simulink model "case4"  (R2024b)
settings: Solver=FixedStepAuto  StartTime=0  StopTime=1  FixedStep=1e-7  RelTol=1e-3
values from neighbouring files (symbols this model uses):
  SG_D_1_D = 0.01056    [IEEE9_case_parameters.m]    (also in case1_parameters.m; case2_parameters.m; case3_parameters.m; case4_parameters.m)
  SG_D_1_EnableSaturation = 0    [IEEE9_case_parameters.m]    (also in case1_parameters.m; case2_parameters.m; case3_parameters.m; case4_parameters.m)
  SG_D_1_f0 = 60    [IEEE9_case_parameters.m]    (also in case1_parameters.m; case2_parameters.m; case3_parameters.m; case4_parameters.m)
  SG_D_1_H = 7.5    [IEEE9_case_parameters.m]    (also in case1_parameters.m; case2_parameters.m; case3_parameters.m; case4_parameters.m)
  SG_D_1_K_A = 20    [IEEE9_case_parameters.m]    (also in case1_parameters.m; case2_parameters.m; case3_parameters.m; case4_parameters.m)
  SG_D_1_K_E = 1.000000e+1    (= 10)    [IEEE9_case_parameters.m]    (also in case1_parameters.m; case2_parameters.m; case3_parameters.m; case4_parameters.m)
  SG_D_1_K_F = 2.363    [IEEE9_case_parameters.m]    (also in case1_parameters.m; case2_parameters.m; case3_parameters.m; case4_parameters.m)
  SG_D_1_K_s = 0.5    [IEEE9_case_parameters.m]    (also in case1_parameters.m = 5; case2_parameters.m = 5; case3_parameters.m = 5; case4_parameters.m = 5)
  SG_D_1_R_a = 0.001088    [IEEE9_case_parameters.m]    (also in case1_parameters.m; case2_parameters.m; case3_parameters.m; case4_parameters.m)
  SG_D_1_S_A = 1    [IEEE9_case_parameters.m]    (also in case1_parameters.m; case2_parameters.m; case3_parameters.m; case4_parameters.m)
  SG_D_1_S_B = 0.103    [IEEE9_case_parameters.m]    (also in case1_parameters.m; case2_parameters.m; case3_parameters.m; case4_parameters.m)
  SG_D_1_S_N = 10.659857    [IEEE9_case_parameters.m]    (also in case1_parameters.m; case2_parameters.m; case3_parameters.m; case4_parameters.m)
  SG_D_1_SpeedPara = 200    [IEEE9_case_parameters.m]    (also in case1_parameters.m; case2_parameters.m; case3_parameters.m; case4_parameters.m)
  SG_D_1_T_0 = 0.720173    [IEEE9_case_parameters.m]    (also in case1_parameters.m = 0.755522; case2_parameters.m = 0.808931; case3_parameters.m = 0.869402; case4_parameters.m = 0.729316)
  SG_D_1_T_1 = 0.3    [IEEE9_case_parameters.m]    (also in case1_parameters.m; case2_parameters.m; case3_parameters.m; case4_parameters.m)
  SG_D_1_T_2 = 0.05    [IEEE9_case_parameters.m]    (also in case1_parameters.m; case2_parameters.m; case3_parameters.m; case4_parameters.m)
  SG_D_1_T_3 = 0.02    [IEEE9_case_parameters.m]    (also in case1_parameters.m; case2_parameters.m; case3_parameters.m; case4_parameters.m)
  SG_D_1_T_4 = 0.005    [IEEE9_case_parameters.m]    (also in case1_parameters.m; case2_parameters.m; case3_parameters.m; case4_parameters.m)
  SG_D_1_T_A = 0.02    [IEEE9_case_parameters.m]    (also in case1_parameters.m; case2_parameters.m; case3_parameters.m; case4_parameters.m)
  SG_D_1_T_dd = 8.000000e+0    (= 8)    [IEEE9_case_parameters.m]    (also in case1_parameters.m; case2_parameters.m; case3_parameters.m; case4_parameters.m)
  SG_D_1_T_ddd = 0.04    [IEEE9_case_parameters.m]    (also in case1_parameters.m; case2_parameters.m; case3_parameters.m; case4_parameters.m)
  SG_D_1_T_E = 0.314    [IEEE9_case_parameters.m]    (also in case1_parameters.m; case2_parameters.m; case3_parameters.m; case4_parameters.m)
  SG_D_1_T_F = 0.35    [IEEE9_case_parameters.m]    (also in case1_parameters.m; case2_parameters.m; case3_parameters.m; case4_parameters.m)
  SG_D_1_T_qd = 0.8    [IEEE9_case_parameters.m]    (also in case1_parameters.m; case2_parameters.m; case3_parameters.m; case4_parameters.m)
  SG_D_1_T_qdd = 0.02    [IEEE9_case_parameters.m]    (also in case1_parameters.m; case2_parameters.m; case3_parameters.m; case4_parameters.m)
  SG_D_1_T_speed = 0.1    [IEEE9_case_parameters.m]    (also in case1_parameters.m = 200; case2_parameters.m = 200; case3_parameters.m = 200; case4_parameters.m = 200)
  SG_D_1_T_w = 0.5    [IEEE9_case_parameters.m]    (also in case1_parameters.m; case2_parameters.m; case3_parameters.m; case4_parameters.m)
  SG_D_1_V_ref = 1.990276    [IEEE9_case_parameters.m]    (also in case1_parameters.m = 2.042296; case2_parameters.m = 2.051388; case3_parameters.m = 2.089584; case4_parameters.m = 2.01845)
  SG_D_1_w_ref = 376.991118    [IEEE9_case_parameters.m]    (also in case1_parameters.m; case2_parameters.m; case3_parameters.m; case4_parameters.m)
  SG_D_1_wb = 6.000000e+1    (= 60)    [IEEE9_case_parameters.m]    (also in case1_parameters.m; case2_parameters.m; case3_parameters.m; case4_parameters.m)
  SG_D_1_x_d = 1.9    [IEEE9_case_parameters.m]    (also in case1_parameters.m; case2_parameters.m; case3_parameters.m; case4_parameters.m)
  SG_D_1_x_dd = 0.302    [IEEE9_case_parameters.m]    (also in case1_parameters.m; case2_parameters.m; case3_parameters.m; case4_parameters.m)
  SG_D_1_x_ddd = 0.204    [IEEE9_case_parameters.m]    (also in case1_parameters.m; case2_parameters.m; case3_parameters.m; case4_parameters.m)
  SG_D_1_x_l = 0.05    [IEEE9_case_parameters.m]    (also in case1_parameters.m; case2_parameters.m; case3_parameters.m; case4_parameters.m)
  SG_D_1_x_q = 1.3    [IEEE9_case_parameters.m]    (also in case1_parameters.m; case2_parameters.m; case3_parameters.m; case4_parameters.m)
  SG_D_1_x_qd = 0.5    [IEEE9_case_parameters.m]    (also in case1_parameters.m; case2_parameters.m; case3_parameters.m; case4_parameters.m)
  SG_D_1_x_qdd = 0.3    [IEEE9_case_parameters.m]    (also in case1_parameters.m; case2_parameters.m; case3_parameters.m; case4_parameters.m)
  SG_D_2_D = 0.02    [IEEE9_case_parameters.m]    (also in case1_parameters.m; case2_parameters.m; case3_parameters.m; case4_parameters.m)
  SG_D_2_EnableSaturation = 0    [IEEE9_case_parameters.m]    (also in case1_parameters.m; case2_parameters.m; case3_parameters.m; case4_parameters.m)
  SG_D_2_f0 = 60    [IEEE9_case_parameters.m]    (also in case1_parameters.m; case2_parameters.m; case3_parameters.m; case4_parameters.m)
  SG_D_2_H = 8.000000e+0    (= 8)    [IEEE9_case_parameters.m]    (also in case1_parameters.m; case2_parameters.m; case3_parameters.m; case4_parameters.m)
  SG_D_2_K_A = 20    [IEEE9_case_parameters.m]    (also in case1_parameters.m; case2_parameters.m; case3_parameters.m; case4_parameters.m)
  SG_D_2_K_E = 1.000000e+1    (= 10)    [IEEE9_case_parameters.m]    (also in case1_parameters.m; case2_parameters.m; case3_parameters.m; case4_parameters.m)
  SG_D_2_K_F = 2.363    [IEEE9_case_parameters.m]    (also in case1_parameters.m; case2_parameters.m; case3_parameters.m; case4_parameters.m)
  SG_D_2_K_s = 0.5    [IEEE9_case_parameters.m]    (also in case1_parameters.m = 4; case2_parameters.m = 4; case3_parameters.m = 4; case4_parameters.m = 4)
  SG_D_2_R_a = 0.001088    [IEEE9_case_parameters.m]    (also in case1_parameters.m; case2_parameters.m; case3_parameters.m; case4_parameters.m)
  SG_D_2_S_A = 1    [IEEE9_case_parameters.m]    (also in case1_parameters.m; case2_parameters.m; case3_parameters.m; case4_parameters.m)
  SG_D_2_S_B = 0.103    [IEEE9_case_parameters.m]    (also in case1_parameters.m; case2_parameters.m; case3_parameters.m; case4_parameters.m)
  SG_D_2_S_N = 10.659857    [IEEE9_case_parameters.m]    (also in case1_parameters.m; case2_parameters.m; case3_parameters.m; case4_parameters.m)
  SG_D_2_SpeedPara = 200    [IEEE9_case_parameters.m]    (also in case1_parameters.m; case2_parameters.m; case3_parameters.m; case4_parameters.m)
  SG_D_2_T_0 = 1.632913    [IEEE9_case_parameters.m]    (also in case1_parameters.m = 1.632925; case2_parameters.m = 1.632915; case3_parameters.m = 1.632914; case4_parameters.m = 1.632927)
  SG_D_2_T_1 = 0.2    [IEEE9_case_parameters.m]    (also in case1_parameters.m; case2_parameters.m; case3_parameters.m; case4_parameters.m)
  SG_D_2_T_2 = 0.05    [IEEE9_case_parameters.m]    (also in case1_parameters.m; case2_parameters.m; case3_parameters.m; case4_parameters.m)
  SG_D_2_T_3 = 0.02    [IEEE9_case_parameters.m]    (also in case1_parameters.m; case2_parameters.m; case3_parameters.m; case4_parameters.m)
  SG_D_2_T_4 = 0.005    [IEEE9_case_parameters.m]    (also in case1_parameters.m; case2_parameters.m; case3_parameters.m; case4_parameters.m)
  SG_D_2_T_A = 0.02    [IEEE9_case_parameters.m]    (also in case1_parameters.m; case2_parameters.m; case3_parameters.m; case4_parameters.m)
  SG_D_2_T_dd = 7.9    [IEEE9_case_parameters.m]    (also in case1_parameters.m; case2_parameters.m; case3_parameters.m; case4_parameters.m)
  SG_D_2_T_ddd = 0.04    [IEEE9_case_parameters.m]    (also in case1_parameters.m; case2_parameters.m; case3_parameters.m; case4_parameters.m)
  SG_D_2_T_E = 0.314    [IEEE9_case_parameters.m]    (also in case1_parameters.m; case2_parameters.m; case3_parameters.m; case4_parameters.m)
  SG_D_2_T_F = 0.35    [IEEE9_case_parameters.m]    (also in case1_parameters.m; case2_parameters.m; case3_parameters.m; case4_parameters.m)
  SG_D_2_T_qd = 0.8    [IEEE9_case_parameters.m]    (also in case1_parameters.m; case2_parameters.m; case3_parameters.m; case4_parameters.m)
  SG_D_2_T_qdd = 0.015    [IEEE9_case_parameters.m]    (also in case1_parameters.m; case2_parameters.m; case3_parameters.m; case4_parameters.m)
  SG_D_2_T_speed = 0.1    [IEEE9_case_parameters.m]    (also in case1_parameters.m = 150; case2_parameters.m = 150; case3_parameters.m = 150; case4_parameters.m = 150)
  SG_D_2_T_w = 0.35    [IEEE9_case_parameters.m]    (also in case1_parameters.m; case2_parameters.m; case3_parameters.m; case4_parameters.m)
  SG_D_2_V_ref = 2.58547    [IEEE9_case_parameters.m]    (also in case1_parameters.m = 2.597896; case2_parameters.m = 2.587136; case3_parameters.m = 2.586042; case4_parameters.m = 2.599679)
  SG_D_2_w_ref = 376.991118    [IEEE9_case_parameters.m]    (also in case1_parameters.m; case2_parameters.m; case3_parameters.m; case4_parameters.m)
  SG_D_2_wb = 6.000000e+1    (= 60)    [IEEE9_case_parameters.m]    (also in case1_parameters.m; case2_parameters.m; case3_parameters.m; case4_parameters.m)
  SG_D_2_x_d = 1.8    [IEEE9_case_parameters.m]    (also in case1_parameters.m; case2_parameters.m; case3_parameters.m; case4_parameters.m)
  SG_D_2_x_dd = 0.302    [IEEE9_case_parameters.m]    (also in case1_parameters.m; case2_parameters.m; case3_parameters.m; case4_parameters.m)
  SG_D_2_x_ddd = 0.204    [IEEE9_case_parameters.m]    (also in case1_parameters.m; case2_parameters.m; case3_parameters.m; case4_parameters.m)
  SG_D_2_x_l = 0.05    [IEEE9_case_parameters.m]    (also in case1_parameters.m; case2_parameters.m; case3_parameters.m; case4_parameters.m)
  SG_D_2_x_q = 1.25    [IEEE9_case_parameters.m]    (also in case1_parameters.m; case2_parameters.m; case3_parameters.m; case4_parameters.m)
  SG_D_2_x_qd = 0.5    [IEEE9_case_parameters.m]    (also in case1_parameters.m; case2_parameters.m; case3_parameters.m; case4_parameters.m)
  SG_D_2_x_qdd = 0.3    [IEEE9_case_parameters.m]    (also in case1_parameters.m; case2_parameters.m; case3_parameters.m; case4_parameters.m)
  SG_D_3_D = 0.02    [IEEE9_case_parameters.m]    (also in case1_parameters.m; case2_parameters.m; case3_parameters.m; case4_parameters.m)
  SG_D_3_EnableSaturation = 0    [IEEE9_case_parameters.m]    (also in case1_parameters.m; case2_parameters.m; case3_parameters.m; case4_parameters.m)
  SG_D_3_f0 = 60    [IEEE9_case_parameters.m]    (also in case1_parameters.m; case2_parameters.m; case3_parameters.m; case4_parameters.m)
  SG_D_3_H = 7.7    [IEEE9_case_parameters.m]    (also in case1_parameters.m; case2_parameters.m; case3_parameters.m; case4_parameters.m)
  SG_D_3_K_A = 20    [IEEE9_case_parameters.m]    (also in case1_parameters.m; case2_parameters.m; case3_parameters.m; case4_parameters.m)
  SG_D_3_K_E = 1.000000e+1    (= 10)    [IEEE9_case_parameters.m]    (also in case1_parameters.m; case2_parameters.m; case3_parameters.m; case4_parameters.m)
  SG_D_3_K_F = 2.363    [IEEE9_case_parameters.m]    (also in case1_parameters.m; case2_parameters.m; case3_parameters.m; case4_parameters.m)
  SG_D_3_K_s = 0.2    [IEEE9_case_parameters.m]    (also in case1_parameters.m = 2; case2_parameters.m = 2; case3_parameters.m = 2; case4_parameters.m = 2)
  SG_D_3_R_a = 0.001088    [IEEE9_case_parameters.m]    (also in case1_parameters.m; case2_parameters.m; case3_parameters.m; case4_parameters.m)
  SG_D_3_S_A = 1    [IEEE9_case_parameters.m]    (also in case1_parameters.m; case2_parameters.m; case3_parameters.m; case4_parameters.m)
  SG_D_3_S_B = 0.103    [IEEE9_case_parameters.m]    (also in case1_parameters.m; case2_parameters.m; case3_parameters.m; case4_parameters.m)
  SG_D_3_S_N = 10.659857    [IEEE9_case_parameters.m]    (also in case1_parameters.m; case2_parameters.m; case3_parameters.m; case4_parameters.m)
  SG_D_3_SpeedPara = 200    [IEEE9_case_parameters.m]    (also in case1_parameters.m; case2_parameters.m; case3_parameters.m; case4_parameters.m)
  SG_D_3_T_0 = 0.850788    [IEEE9_case_parameters.m]    (also in case1_parameters.m = 0.850786; case2_parameters.m = 0.850787; case3_parameters.m; case4_parameters.m = 0.850786)
  SG_D_3_T_1 = 0.2    [IEEE9_case_parameters.m]    (also in case1_parameters.m; case2_parameters.m; case3_parameters.m; case4_parameters.m)
  SG_D_3_T_2 = 0.05    [IEEE9_case_parameters.m]    (also in case1_parameters.m; case2_parameters.m; case3_parameters.m; case4_parameters.m)
  SG_D_3_T_3 = 0.02    [IEEE9_case_parameters.m]    (also in case1_parameters.m; case2_parameters.m; case3_parameters.m; case4_parameters.m)
  SG_D_3_T_4 = 0.005    [IEEE9_case_parameters.m]    (also in case1_parameters.m; case2_parameters.m; case3_parameters.m; case4_parameters.m)
  SG_D_3_T_A = 0.02    [IEEE9_case_parameters.m]    (also in case1_parameters.m; case2_parameters.m; case3_parameters.m; case4_parameters.m)
  SG_D_3_T_dd = 8.1    [IEEE9_case_parameters.m]    (also in case1_parameters.m; case2_parameters.m; case3_parameters.m; case4_parameters.m)
  SG_D_3_T_ddd = 0.04    [IEEE9_case_parameters.m]    (also in case1_parameters.m; case2_parameters.m; case3_parameters.m; case4_parameters.m)
  SG_D_3_T_E = 0.314    [IEEE9_case_parameters.m]    (also in case1_parameters.m; case2_parameters.m; case3_parameters.m; case4_parameters.m)
  SG_D_3_T_F = 0.35    [IEEE9_case_parameters.m]    (also in case1_parameters.m; case2_parameters.m; case3_parameters.m; case4_parameters.m)
  SG_D_3_T_qd = 0.8    [IEEE9_case_parameters.m]    (also in case1_parameters.m; case2_parameters.m; case3_parameters.m; case4_parameters.m)
  SG_D_3_T_qdd = 0.015    [IEEE9_case_parameters.m]    (also in case1_parameters.m; case2_parameters.m; case3_parameters.m; case4_parameters.m)
  SG_D_3_T_speed = 0.1    [IEEE9_case_parameters.m]    (also in case1_parameters.m = 180; case2_parameters.m = 180; case3_parameters.m = 180; case4_parameters.m = 180)
  SG_D_3_T_w = 0.4    [IEEE9_case_parameters.m]    (also in case1_parameters.m; case2_parameters.m; case3_parameters.m; case4_parameters.m)
  SG_D_3_V_ref = 1.892727    [IEEE9_case_parameters.m]    (also in case1_parameters.m = 1.906439; case2_parameters.m = 1.895535; case3_parameters.m = 1.892105; case4_parameters.m = 1.906598)
  SG_D_3_w_ref = 376.991118    [IEEE9_case_parameters.m]    (also in case1_parameters.m; case2_parameters.m; case3_parameters.m; case4_parameters.m)
  SG_D_3_wb = 6.000000e+1    (= 60)    [IEEE9_case_parameters.m]    (also in case1_parameters.m; case2_parameters.m; case3_parameters.m; case4_parameters.m)
  SG_D_3_x_d = 1.85    [IEEE9_case_parameters.m]    (also in case1_parameters.m; case2_parameters.m; case3_parameters.m; case4_parameters.m)
  SG_D_3_x_dd = 0.302    [IEEE9_case_parameters.m]    (also in case1_parameters.m; case2_parameters.m; case3_parameters.m; case4_parameters.m)
  SG_D_3_x_ddd = 0.204    [IEEE9_case_parameters.m]    (also in case1_parameters.m; case2_parameters.m; case3_parameters.m; case4_parameters.m)
  SG_D_3_x_l = 0.05    [IEEE9_case_parameters.m]    (also in case1_parameters.m; case2_parameters.m; case3_parameters.m; case4_parameters.m)
  SG_D_3_x_q = 1.2    [IEEE9_case_parameters.m]    (also in case1_parameters.m; case2_parameters.m; case3_parameters.m; case4_parameters.m)
  SG_D_3_x_qd = 0.5    [IEEE9_case_parameters.m]    (also in case1_parameters.m; case2_parameters.m; case3_parameters.m; case4_parameters.m)
  SG_D_3_x_qdd = 0.3    [IEEE9_case_parameters.m]    (also in case1_parameters.m; case2_parameters.m; case3_parameters.m; case4_parameters.m)
(part 1 of 12)
settings Model: Creator=Greg  LastModifiedBy=Greg

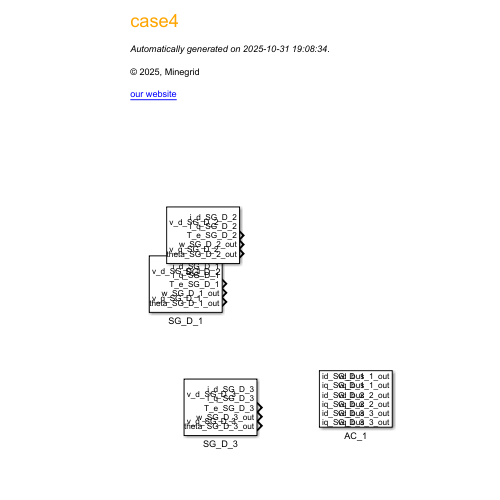
[thumbnail: Simulink's stored preview of the top-level diagram]
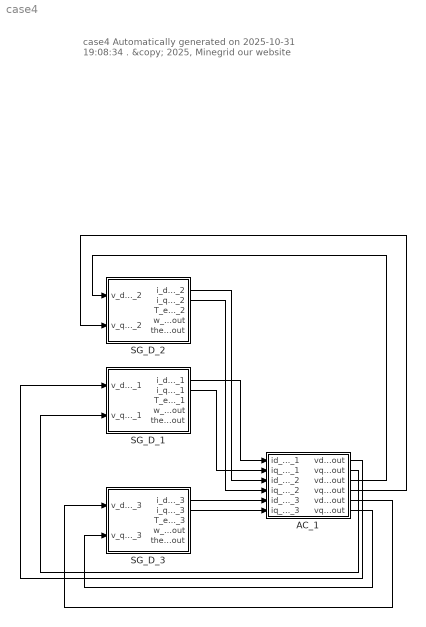
== system case4 ==
  note: case4
      | Automatically generated on 2025-10-31 19:08:34 .
      | &copy; 2025, Minegrid
      | our website
  AC_1 : Subsystem  mask(AC_1){}
      mask help: Parameters Interface of AC_1
  SG_D_1 : Subsystem  mask(SG_D_1){T_0=SG_D_1_T_0, w_ref=SG_D_1_w_ref, V_ref=SG_D_1_V_ref, x_d=SG_D_1_x_d, x_dd=SG_D_1_x_dd, x_ddd=SG_D_1_x_ddd, x_q=SG_D_1_x_q, x_qd=SG_D_1_x_qd, x_qdd=SG_D_1_x_qdd, x_l=SG_D_1_x_l, R_a=SG_D_1_R_a, T_dd=SG_D_1_T_dd, T_ddd=SG_D_1_T_ddd, T_qd=SG_D_1_T_qd, T_qdd=SG_D_1_T_qdd, H=SG_D_1_H, D=SG_D_1_D, SpeedPara=SG_D_1_SpeedPara, K_A=SG_D_1_K_A, EnableSaturation=SG_D_1_EnableSaturation, f0=SG_D_1_f0, T_speed=SG_D_1_T_speed, T_E=SG_D_1_T_E, T_A=SG_D_1_T_A, T_F=SG_D_1_T_F, K_E=SG_D_1_K_E, K_F=SG_D_1_K_F, K_s=SG_D_1_K_s, T_1=SG_D_1_T_1, T_2=SG_D_1_T_2, T_3=SG_D_1_T_3, T_4=SG_D_1_T_4, T_w=SG_D_1_T_w, wb=SG_D_1_wb, S_A=SG_D_1_S_A, S_B=SG_D_1_S_B, S_N=SG_D_1_S_N}
      mask help: Parameters Interface of SG_D_1
  SG_D_2 : Subsystem  mask(SG_D_2){T_0=SG_D_2_T_0, w_ref=SG_D_2_w_ref, V_ref=SG_D_2_V_ref, x_d=SG_D_2_x_d, x_dd=SG_D_2_x_dd, x_ddd=SG_D_2_x_ddd, x_q=SG_D_2_x_q, x_qd=SG_D_2_x_qd, x_qdd=SG_D_2_x_qdd, x_l=SG_D_2_x_l, R_a=SG_D_2_R_a, T_dd=SG_D_2_T_dd, T_ddd=SG_D_2_T_ddd, T_qd=SG_D_2_T_qd, T_qdd=SG_D_2_T_qdd, H=SG_D_2_H, D=SG_D_2_D, SpeedPara=SG_D_2_SpeedPara, K_A=SG_D_2_K_A, EnableSaturation=SG_D_2_EnableSaturation, f0=SG_D_2_f0, T_speed=SG_D_2_T_speed, T_E=SG_D_2_T_E, T_A=SG_D_2_T_A, T_F=SG_D_2_T_F, K_E=SG_D_2_K_E, K_F=SG_D_2_K_F, K_s=SG_D_2_K_s, T_1=SG_D_2_T_1, T_2=SG_D_2_T_2, T_3=SG_D_2_T_3, T_4=SG_D_2_T_4, T_w=SG_D_2_T_w, wb=SG_D_2_wb, S_A=SG_D_2_S_A, S_B=SG_D_2_S_B, S_N=SG_D_2_S_N}
      mask help: Parameters Interface of SG_D_2
  SG_D_3 : Subsystem  mask(SG_D_3){T_0=SG_D_3_T_0, w_ref=SG_D_3_w_ref, V_ref=SG_D_3_V_ref, x_d=SG_D_3_x_d, x_dd=SG_D_3_x_dd, x_ddd=SG_D_3_x_ddd, x_q=SG_D_3_x_q, x_qd=SG_D_3_x_qd, x_qdd=SG_D_3_x_qdd, x_l=SG_D_3_x_l, R_a=SG_D_3_R_a, T_dd=SG_D_3_T_dd, T_ddd=SG_D_3_T_ddd, T_qd=SG_D_3_T_qd, T_qdd=SG_D_3_T_qdd, H=SG_D_3_H, D=SG_D_3_D, SpeedPara=SG_D_3_SpeedPara, K_A=SG_D_3_K_A, EnableSaturation=SG_D_3_EnableSaturation, f0=SG_D_3_f0, T_speed=SG_D_3_T_speed, T_E=SG_D_3_T_E, T_A=SG_D_3_T_A, T_F=SG_D_3_T_F, K_E=SG_D_3_K_E, K_F=SG_D_3_K_F, K_s=SG_D_3_K_s, T_1=SG_D_3_T_1, T_2=SG_D_3_T_2, T_3=SG_D_3_T_3, T_4=SG_D_3_T_4, T_w=SG_D_3_T_w, wb=SG_D_3_wb, S_A=SG_D_3_S_A, S_B=SG_D_3_S_B, S_N=SG_D_3_S_N}
      mask help: Parameters Interface of SG_D_3
  wires:
  SG_D_2/1(i_d_SG_D_2) -> AC_1/3(id_SG_D_2)
  SG_D_1/2(i_q_SG_D_1) -> AC_1/2(iq_SG_D_1)
  SG_D_1/1(i_d_SG_D_1) -> AC_1/1(id_SG_D_1)
  SG_D_2/2(i_q_SG_D_2) -> AC_1/4(iq_SG_D_2)
  AC_1/1(vd_bus_1_out) -> SG_D_1/1(v_d_SG_D_1)
  SG_D_3/1(i_d_SG_D_3) -> AC_1/5(id_SG_D_3)
  AC_1/2(vq_bus_1_out) -> SG_D_1/2(v_q_SG_D_1)
  SG_D_3/2(i_q_SG_D_3) -> AC_1/6(iq_SG_D_3)
  AC_1/3(vd_bus_2_out) -> SG_D_2/1(v_d_SG_D_2)
  AC_1/4(vq_bus_2_out) -> SG_D_2/2(v_q_SG_D_2)
  AC_1/5(vd_bus_3_out) -> SG_D_3/1(v_d_SG_D_3)
  AC_1/6(vq_bus_3_out) -> SG_D_3/2(v_q_SG_D_3)

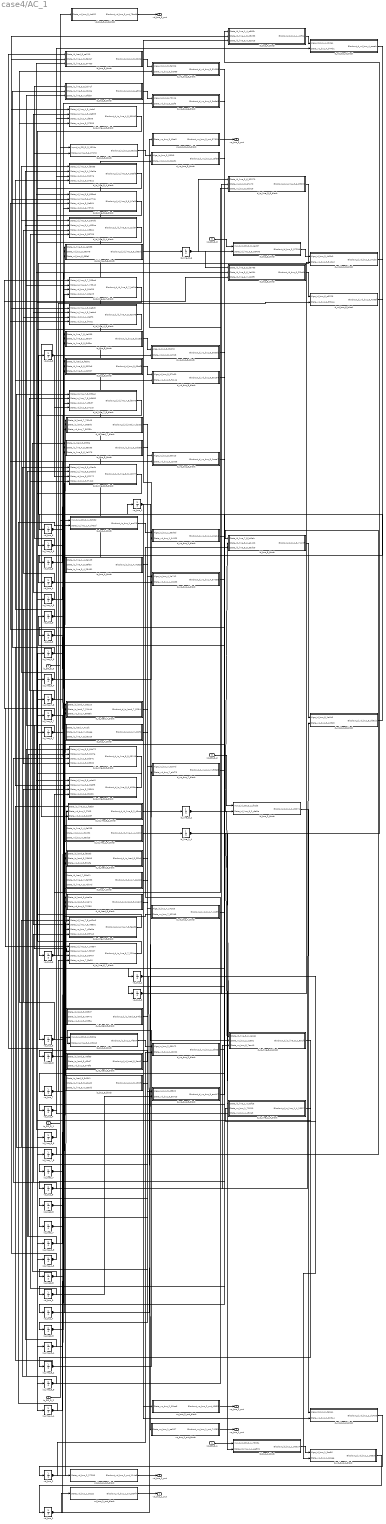
== system case4/AC_1 ==
  id_SG_D_1 : Inport
  iq_SG_D_1 : Inport  Port=2
  id_SG_D_2 : Inport  Port=3
  iq_SG_D_2 : Inport  Port=4
  id_SG_D_3 : Inport  Port=5
  iq_SG_D_3 : Inport  Port=6
  d_id_line_1_4_block : Subsystem
  d_id_line_3_6_block : Subsystem
  d_id_line_4_5_block : Subsystem
  d_id_line_5_6_block : Subsystem
  d_id_line_6_7_block : Subsystem
  d_id_line_7_8_block : Subsystem
  d_id_line_8_2_block : Subsystem
  d_id_line_8_9_block : Subsystem
  d_id_line_9_4_block : Subsystem
  d_id_load_5_block : Subsystem
  d_id_load_7_block : Subsystem
  d_id_load_9_block : Subsystem
  d_iq_line_1_4_block : Subsystem
  d_iq_line_3_6_block : Subsystem
  d_iq_line_4_5_block : Subsystem
  d_iq_line_5_6_block : Subsystem
  d_iq_line_6_7_block : Subsystem
  d_iq_line_7_8_block : Subsystem
  d_iq_line_8_2_block : Subsystem
  d_iq_line_8_9_block : Subsystem
  d_iq_line_9_4_block : Subsystem
  d_iq_load_5_block : Subsystem
  d_iq_load_7_block : Subsystem
  d_iq_load_9_block : Subsystem
  d_vd_bus_1_block : Subsystem
  d_vd_bus_2_block : Subsystem
  d_vd_bus_3_block : Subsystem
  d_vd_bus_4_block : Subsystem
  d_vd_bus_5_block : Subsystem
  d_vd_bus_6_block : Subsystem
  d_vd_bus_7_block : Subsystem
  d_vd_bus_8_block : Subsystem
  d_vd_bus_9_block : Subsystem
  d_vq_bus_1_block : Subsystem
  d_vq_bus_2_block : Subsystem
  d_vq_bus_3_block : Subsystem
  d_vq_bus_4_block : Subsystem
  d_vq_bus_5_block : Subsystem
  d_vq_bus_6_block : Subsystem
  d_vq_bus_7_block : Subsystem
  d_vq_bus_8_block : Subsystem
  d_vq_bus_9_block : Subsystem
  id_bus_1_block : Subsystem
  id_bus_2_block : Subsystem
  id_bus_3_block : Subsystem
  id_bus_4_block : Subsystem
  id_bus_5_block : Subsystem
  id_bus_6_block : Subsystem
  id_bus_7_block : Subsystem
  id_bus_8_block : Subsystem
  id_bus_9_block : Subsystem
  id_line_1_4 : Integrator  InitialCondition=0.7287
  id_line_3_6 : Integrator  InitialCondition=0.846
  id_line_4_5 : Integrator  InitialCondition=0.3118
  id_line_5_6 : Integrator  InitialCondition=-0.6087
  id_line_6_7 : Integrator  InitialCondition=0.247
  id_line_7_8 : Integrator  InitialCondition=-0.7758
  id_line_8_2 : Integrator  InitialCondition=-1.6368
  id_line_8_9 : Integrator  InitialCondition=0.8765
  id_line_9_4 : Integrator  InitialCondition=-0.4095
  id_load_5 : Integrator  InitialCondition=0.9018637525113781
  id_load_7 : Integrator  InitialCondition=1.0245286683766606
  id_load_9 : Integrator  InitialCondition=1.2674774745630744
  iq_bus_1_block : Subsystem
  iq_bus_2_block : Subsystem
  iq_bus_3_block : Subsystem
  iq_bus_4_block : Subsystem
  iq_bus_5_block : Subsystem
  iq_bus_6_block : Subsystem
  iq_bus_7_block : Subsystem
  iq_bus_8_block : Subsystem
  iq_bus_9_block : Subsystem
  iq_line_1_4 : Integrator  InitialCondition=-0.272
  iq_line_3_6 : Integrator  InitialCondition=0.0827
  iq_line_4_5 : Integrator  InitialCondition=-0.0945
  iq_line_5_6 : Integrator  InitialCondition=0.0478
  iq_line_6_7 : Integrator  InitialCondition=-0.1534
  iq_line_7_8 : Integrator  InitialCondition=0.0347
  iq_line_8_2 : Integrator  InitialCondition=-0.1054
  iq_line_8_9 : Integrator  InitialCondition=-0.0855
  iq_line_9_4 : Integrator  InitialCondition=0.3418
  iq_load_5 : Integrator  InitialCondition=-0.39236911133703173
  iq_load_7 : Integrator  InitialCondition=-0.3639221819066319
  iq_load_9 : Integrator  InitialCondition=-0.6559840473105716
  vd_bus_1 : Integrator  InitialCondition=1.0
  vd_bus_1_out_block : Subsystem
  vd_bus_2 : Integrator  InitialCondition=0.9845573566855935
  vd_bus_2_out_block : Subsystem
  vd_bus_3 : Integrator  InitialCondition=0.9962979583371808
  vd_bus_3_out_block : Subsystem
  vd_bus_4 : Integrator  InitialCondition=0.9836041408890515
  vd_bus_5 : Integrator  InitialCondition=0.969229495709966
  vd_bus_6 : Integrator  InitialCondition=1.0013698000105777
  vd_bus_7 : Integrator  InitialCondition=0.9822666807981633
  vd_bus_8 : Integrator  InitialCondition=0.9914484628723825
  vd_bus_9 : Integrator  InitialCondition=0.9491262958289386
  vq_bus_1 : Integrator  InitialCondition=0.0
  vq_bus_1_out_block : Subsystem
  vq_bus_2 : Integrator  InitialCondition=0.1750623071831195
  vq_bus_2_out_block : Subsystem
  vq_bus_3 : Integrator  InitialCondition=0.08596730897943144
  vq_bus_3_out_block : Subsystem
  vq_bus_4 : Integrator  InitialCondition=-0.043919709875534375
  vq_bus_5 : Integrator  InitialCondition=-0.07234036863293895
  vq_bus_6 : Integrator  InitialCondition=0.0340882018123715
  vq_bus_7 : Integrator  InitialCondition=0.009853330044675679
  vq_bus_8 : Integrator  InitialCondition=0.06800966582463833
  vq_bus_9 : Integrator  InitialCondition=-0.07694083587590034
  vd_bus_1_out : Outport
  vq_bus_1_out : Outport  Port=2
  vd_bus_2_out : Outport  Port=3
  vq_bus_2_out : Outport  Port=4
  vd_bus_3_out : Outport  Port=5
  vq_bus_3_out : Outport  Port=6
  wires:
  vq_bus_2_out_block/1(Blockout_vq_bus_2_out_4fd53) -> vq_bus_2_out/1
  d_id_line_1_4_block/1(Blockout_d_id_line_1_4_c12b1) -> id_line_1_4/1
  iq_SG_D_3/1 -> iq_bus_3_block/1(Input_iq_SG_D_3_132dc)
  id_SG_D_2/1 -> id_bus_2_block/1(Input_id_SG_D_2_fbcda)
  d_vd_bus_4_block/1(Blockout_d_vd_bus_4_acceb) -> vd_bus_4/1
  id_SG_D_3/1 -> id_bus_3_block/1(Input_id_SG_D_3_1ed07)
  d_iq_line_8_2_block/1(Blockout_d_iq_line_8_2_851f9) -> iq_line_8_2/1
  vd_bus_3_out_block/1(Blockout_vd_bus_3_out_78edb) -> vd_bus_3_out/1
  vq_bus_1/1 -> d_iq_line_1_4_block/2(State_vq_bus_1_71810), d_vd_bus_1_block/2(State_vq_bus_1_c46ee), vq_bus_1_out_block/1(State_vq_bus_1_ae207)
  id_bus_5_block/1(Blockout_id_bus_5_00d6f) -> d_vd_bus_5_block/1(Alge_id_bus_5_5a326)
  iq_bus_4_block/1(Blockout_iq_bus_4_4c52a) -> d_vq_bus_4_block/1(Alge_iq_bus_4_1a742)
  id_line_6_7/1 -> id_bus_6_block/3(State_id_line_6_7_1ddf3), d_iq_line_6_7_block/1(State_id_line_6_7_c49e4), d_id_line_6_7_block/1(State_id_line_6_7_205ed), id_bus_7_block/2(State_id_line_6_7_3a993)
  id_bus_2_block/1(Blockout_id_bus_2_d0074) -> d_vd_bus_2_block/1(Alge_id_bus_2_da6a4)
  iq_SG_D_2/1 -> iq_bus_2_block/1(Input_iq_SG_D_2_5cb3e)
  d_id_line_7_8_block/1(Blockout_d_id_line_7_8_fa870) -> id_line_7_8/1
  id_bus_9_block/1(Blockout_id_bus_9_09ef3) -> d_vd_bus_9_block/1(Alge_id_bus_9_57b60)
  iq_SG_D_1/1 -> iq_bus_1_block/1(Input_iq_SG_D_1_3d98d)
  id_line_4_5/1 -> id_bus_4_block/2(State_id_line_4_5_25293), d_id_line_4_5_block/1(State_id_line_4_5_be8c5), d_iq_line_4_5_block/1(State_id_line_4_5_4cdcf), id_bus_5_block/2(State_id_line_4_5_86da7)
  id_bus_6_block/1(Blockout_id_bus_6_23bdb) -> d_vd_bus_6_block/1(Alge_id_bus_6_a9226)
  iq_bus_9_block/1(Blockout_iq_bus_9_13bf1) -> d_vq_bus_9_block/1(Alge_iq_bus_9_c8820)
  d_iq_load_7_block/1(Blockout_d_iq_load_7_52844) -> iq_load_7/1
  id_SG_D_1/1 -> id_bus_1_block/1(Input_id_SG_D_1_73334)
  vq_bus_3_out_block/1(Blockout_vq_bus_3_out_5791b) -> vq_bus_3_out/1
  iq_bus_8_block/1(Blockout_iq_bus_8_d2159) -> d_vq_bus_8_block/1(Alge_iq_bus_8_9b29c)
  iq_line_5_6/1 -> d_iq_line_5_6_block/2(State_iq_line_5_6_96bf5), iq_bus_5_block/3(State_iq_line_5_6_1a976), iq_bus_6_block/2(State_iq_line_5_6_2bdce), d_id_line_5_6_block/2(State_iq_line_5_6_e77ce)
  id_bus_3_block/1(Blockout_id_bus_3_9729d) -> d_vd_bus_3_block/1(Alge_id_bus_3_4d9b0)
  id_bus_8_block/1(Blockout_id_bus_8_7113f) -> d_vd_bus_8_block/1(Alge_id_bus_8_1a6c3)
  iq_load_7/1 -> d_iq_load_7_block/2(State_iq_load_7_2144d), iq_bus_7_block/1(State_iq_load_7_41cfc), d_id_load_7_block/2(State_iq_load_7_8050b)
  id_bus_7_block/1(Blockout_id_bus_7_de2dd) -> d_vd_bus_7_block/1(Alge_id_bus_7_14163)
  vq_bus_8/1 -> d_iq_line_7_8_block/4(State_vq_bus_8_897ad), d_iq_line_8_2_block/3(State_vq_bus_8_7ea40), d_vd_bus_8_block/2(State_vq_bus_8_4d3d0), d_iq_line_8_9_block/3(State_vq_bus_8_6d34c)
  iq_bus_7_block/1(Blockout_iq_bus_7_c21f1) -> d_vq_bus_7_block/1(Alge_iq_bus_7_a187d)
  d_id_load_7_block/1(Blockout_d_id_load_7_d2cec) -> id_load_7/1
  iq_bus_6_block/1(Blockout_iq_bus_6_e334f) -> d_vq_bus_6_block/1(Alge_iq_bus_6_7b11a)
  iq_bus_5_block/1(Blockout_iq_bus_5_1eb56) -> d_vq_bus_5_block/1(Alge_iq_bus_5_60a13)
  vd_bus_2_out_block/1(Blockout_vd_bus_2_out_114e8) -> vd_bus_2_out/1
  d_iq_line_7_8_block/1(Blockout_d_iq_line_7_8_fee52) -> iq_line_7_8/1
  iq_bus_3_block/1(Blockout_iq_bus_3_0e2bc) -> d_vq_bus_3_block/1(Alge_iq_bus_3_05f49)
  id_load_9/1 -> d_iq_load_9_block/1(State_id_load_9_3092f), id_bus_9_block/1(State_id_load_9_f6d0c), d_id_load_9_block/1(State_id_load_9_aba5e)
  id_bus_4_block/1(Blockout_id_bus_4_42f24) -> d_vd_bus_4_block/1(Alge_id_bus_4_12de4)
  vd_bus_1_out_block/1(Blockout_vd_bus_1_out_8e4f7) -> vd_bus_1_out/1
  vq_bus_1_out_block/1(Blockout_vq_bus_1_out_74281) -> vq_bus_1_out/1
  d_vd_bus_3_block/1(Blockout_d_vd_bus_3_c41ba) -> vd_bus_3/1
  iq_bus_2_block/1(Blockout_iq_bus_2_7f564) -> d_vq_bus_2_block/1(Alge_iq_bus_2_66b72)
  iq_line_8_2/1 -> iq_bus_2_block/2(State_iq_line_8_2_0316d), iq_bus_8_block/2(State_iq_line_8_2_39c57), d_id_line_8_2_block/1(State_iq_line_8_2_fc8b9)
  iq_bus_1_block/1(Blockout_iq_bus_1_acc76) -> d_vq_bus_1_block/1(Alge_iq_bus_1_5ed0d)
  d_vq_bus_7_block/1(Blockout_d_vq_bus_7_f8968) -> vq_bus_7/1
  vd_bus_5/1 -> d_vq_bus_5_block/2(State_vd_bus_5_c20a6), d_id_line_4_5_block/4(State_vd_bus_5_f7ecc), d_id_line_5_6_block/3(State_vd_bus_5_0e564), d_id_load_5_block/3(State_vd_bus_5_078f0)
  id_bus_1_block/1(Blockout_id_bus_1_00a24) -> d_vd_bus_1_block/1(Alge_id_bus_1_3cc56)
  d_vd_bus_5_block/1(Blockout_d_vd_bus_5_51008) -> vd_bus_5/1
  d_id_line_3_6_block/1(Blockout_d_id_line_3_6_d53d7) -> id_line_3_6/1
  d_id_line_6_7_block/1(Blockout_d_id_line_6_7_bd2cf) -> id_line_6_7/1
  d_id_line_8_2_block/1(Blockout_d_id_line_8_2_d5ea8) -> id_line_8_2/1
  id_line_3_6/1 -> id_bus_3_block/2(State_id_line_3_6_05496), id_bus_6_block/1(State_id_line_3_6_de78e), d_iq_line_3_6_block/1(State_id_line_3_6_92370)
  id_line_7_8/1 -> id_bus_8_block/1(State_id_line_7_8_b4fab), d_id_line_7_8_block/1(State_id_line_7_8_95bec), id_bus_7_block/3(State_id_line_7_8_7bb7d), d_iq_line_7_8_block/1(State_id_line_7_8_e42a6)
  d_iq_load_9_block/1(Blockout_d_iq_load_9_a4f21) -> iq_load_9/1
  d_id_line_9_4_block/1(Blockout_d_id_line_9_4_11d37) -> id_line_9_4/1
  vq_bus_5/1 -> d_vd_bus_5_block/2(State_vq_bus_5_bc989), d_iq_line_4_5_block/4(State_vq_bus_5_37393), d_iq_line_5_6_block/3(State_vq_bus_5_29364), d_iq_load_5_block/3(State_vq_bus_5_534fe)
  d_iq_line_5_6_block/1(Blockout_d_iq_line_5_6_b33bc) -> iq_line_5_6/1
  iq_line_1_4/1 -> iq_bus_1_block/2(State_iq_line_1_4_d402f), iq_bus_4_block/1(State_iq_line_1_4_0e1d9), d_id_line_1_4_block/1(State_iq_line_1_4_0e235)
  d_vd_bus_9_block/1(Blockout_d_vd_bus_9_6a164) -> vd_bus_9/1
  vq_bus_9/1 -> d_vd_bus_9_block/2(State_vq_bus_9_f1146), d_iq_load_9_block/3(State_vq_bus_9_4335e), d_iq_line_8_9_block/4(State_vq_bus_9_b3300), d_iq_line_9_4_block/4(State_vq_bus_9_e7522)
  iq_load_9/1 -> d_id_load_9_block/2(State_iq_load_9_24674), d_iq_load_9_block/2(State_iq_load_9_43472), iq_bus_9_block/1(State_iq_load_9_5d541)
  d_vq_bus_4_block/1(Blockout_d_vq_bus_4_57ae8) -> vq_bus_4/1
  d_vq_bus_3_block/1(Blockout_d_vq_bus_3_13f3e) -> vq_bus_3/1
  d_vq_bus_1_block/1(Blockout_d_vq_bus_1_40e24) -> vq_bus_1/1
  id_line_8_9/1 -> id_bus_8_block/3(State_id_line_8_9_3adb9), d_iq_line_8_9_block/1(State_id_line_8_9_6dd72), id_bus_9_block/2(State_id_line_8_9_502b6), d_id_line_8_9_block/1(State_id_line_8_9_d1adb)
  iq_line_9_4/1 -> d_id_line_9_4_block/2(State_iq_line_9_4_d03ba), d_iq_line_9_4_block/2(State_iq_line_9_4_10a5e), iq_bus_4_block/3(State_iq_line_9_4_28481), iq_bus_9_block/3(State_iq_line_9_4_ce0dd)
  vd_bus_4/1 -> d_id_line_1_4_block/3(State_vd_bus_4_3ed23), d_id_line_4_5_block/3(State_vd_bus_4_de2fb), d_vq_bus_4_block/2(State_vd_bus_4_18c33), d_id_line_9_4_block/3(State_vd_bus_4_18861)
  id_line_9_4/1 -> id_bus_4_block/3(State_id_line_9_4_32915), d_id_line_9_4_block/1(State_id_line_9_4_a375b), d_iq_line_9_4_block/1(State_id_line_9_4_f5685), id_bus_9_block/3(State_id_line_9_4_0d307)
  iq_line_8_9/1 -> d_id_line_8_9_block/2(State_iq_line_8_9_5adad), d_iq_line_8_9_block/2(State_iq_line_8_9_3cc7e), iq_bus_8_block/3(State_iq_line_8_9_fb39e), iq_bus_9_block/2(State_iq_line_8_9_a2ec0)
  vd_bus_9/1 -> d_id_line_9_4_block/4(State_vd_bus_9_95759), d_vq_bus_9_block/2(State_vd_bus_9_5e7c3), d_id_line_8_9_block/4(State_vd_bus_9_f74b0), d_id_load_9_block/3(State_vd_bus_9_72280)
  id_line_8_2/1 -> d_iq_line_8_2_block/1(State_id_line_8_2_1a66c), id_bus_2_block/2(State_id_line_8_2_cfe5e), id_bus_8_block/2(State_id_line_8_2_e242b)
  iq_line_7_8/1 -> d_id_line_7_8_block/2(State_iq_line_7_8_b5b80), d_iq_line_7_8_block/2(State_iq_line_7_8_485ac), iq_bus_7_block/3(State_iq_line_7_8_b62c9), iq_bus_8_block/1(State_iq_line_7_8_4e039)
  vd_bus_8/1 -> d_id_line_7_8_block/4(State_vd_bus_8_a71c0), d_id_line_8_2_block/3(State_vd_bus_8_bcd3f), d_id_line_8_9_block/3(State_vd_bus_8_62172), d_vq_bus_8_block/2(State_vd_bus_8_14918)
  iq_line_6_7/1 -> d_id_line_6_7_block/2(State_iq_line_6_7_7334d), d_iq_line_6_7_block/2(State_iq_line_6_7_f03d7), iq_bus_6_block/3(State_iq_line_6_7_0fdb9), iq_bus_7_block/2(State_iq_line_6_7_12eee)
  iq_line_4_5/1 -> d_id_line_4_5_block/2(State_iq_line_4_5_1edad), d_iq_line_4_5_block/2(State_iq_line_4_5_de839), iq_bus_4_block/2(State_iq_line_4_5_08faa), iq_bus_5_block/2(State_iq_line_4_5_55a5a)
  vd_bus_2/1 -> d_vq_bus_2_block/2(State_vd_bus_2_c0202), vd_bus_2_out_block/1(State_vd_bus_2_27286), d_id_line_8_2_block/2(State_vd_bus_2_f74f3)
  id_line_5_6/1 -> d_id_line_5_6_block/1(State_id_line_5_6_669ed), d_iq_line_5_6_block/1(State_id_line_5_6_cde43), id_bus_5_block/3(State_id_line_5_6_37460), id_bus_6_block/2(State_id_line_5_6_1a694)
  iq_line_3_6/1 -> d_id_line_3_6_block/1(State_iq_line_3_6_4e988), iq_bus_3_block/2(State_iq_line_3_6_0719c), iq_bus_6_block/1(State_iq_line_3_6_bd71f)
  vd_bus_3/1 -> vd_bus_3_out_block/1(State_vd_bus_3_4cb32), d_id_line_3_6_block/2(State_vd_bus_3_a6578), d_vq_bus_3_block/2(State_vd_bus_3_0de91)
  id_line_1_4/1 -> d_iq_line_1_4_block/1(State_id_line_1_4_0dfc6), id_bus_1_block/2(State_id_line_1_4_ee531), id_bus_4_block/1(State_id_line_1_4_a86fb)
  id_load_7/1 -> d_id_load_7_block/1(State_id_load_7_751d5), d_iq_load_7_block/1(State_id_load_7_6612a), id_bus_7_block/1(State_id_load_7_08a11)
  iq_load_5/1 -> d_id_load_5_block/2(State_iq_load_5_dfbd7), d_iq_load_5_block/2(State_iq_load_5_28b96), iq_bus_5_block/1(State_iq_load_5_b9fd6)
  id_load_5/1 -> d_id_load_5_block/1(State_id_load_5_45f50), d_iq_load_5_block/1(State_id_load_5_f6e5b), id_bus_5_block/1(State_id_load_5_ce210)
  vd_bus_1/1 -> d_id_line_1_4_block/2(State_vd_bus_1_91d32), vd_bus_1_out_block/1(State_vd_bus_1_6cc2c), d_vq_bus_1_block/2(State_vd_bus_1_041f3)
  vd_bus_7/1 -> d_vq_bus_7_block/2(State_vd_bus_7_abf75), d_id_load_7_block/3(State_vd_bus_7_9625b), d_id_line_6_7_block/4(State_vd_bus_7_0da25), d_id_line_7_8_block/3(State_vd_bus_7_dfa37)
  vq_bus_7/1 -> d_vd_bus_7_block/2(State_vq_bus_7_922d5), d_iq_load_7_block/3(State_vq_bus_7_6865b), d_iq_line_6_7_block/4(State_vq_bus_7_ffa00), d_iq_line_7_8_block/3(State_vq_bus_7_d0e8e)
  vd_bus_6/1 -> d_vq_bus_6_block/2(State_vd_bus_6_cccf8), d_id_line_5_6_block/4(State_vd_bus_6_757cb), d_id_line_3_6_block/3(State_vd_bus_6_66fef), d_id_line_6_7_block/3(State_vd_bus_6_54d39)
  vq_bus_6/1 -> d_iq_line_3_6_block/3(State_vq_bus_6_0d319), d_vd_bus_6_block/2(State_vq_bus_6_35b4a), d_iq_line_5_6_block/4(State_vq_bus_6_3bcbb), d_iq_line_6_7_block/3(State_vq_bus_6_ae467)
  vq_bus_4/1 -> d_vd_bus_4_block/2(State_vq_bus_4_d44b1), d_iq_line_1_4_block/3(State_vq_bus_4_452a3), d_iq_line_4_5_block/3(State_vq_bus_4_cf608), d_iq_line_9_4_block/3(State_vq_bus_4_9407e)
  vq_bus_3/1 -> d_iq_line_3_6_block/2(State_vq_bus_3_67a70), d_vd_bus_3_block/2(State_vq_bus_3_54d4d), vq_bus_3_out_block/1(State_vq_bus_3_4fca5)
  vq_bus_2/1 -> d_iq_line_8_2_block/2(State_vq_bus_2_c1e81), d_vd_bus_2_block/2(State_vq_bus_2_02344), vq_bus_2_out_block/1(State_vq_bus_2_03ca6)
  d_vq_bus_9_block/1(Blockout_d_vq_bus_9_ae447) -> vq_bus_9/1
  d_iq_line_9_4_block/1(Blockout_d_iq_line_9_4_8eaf6) -> iq_line_9_4/1
  d_id_line_4_5_block/1(Blockout_d_id_line_4_5_92e48) -> id_line_4_5/1
  d_iq_line_3_6_block/1(Blockout_d_iq_line_3_6_89b36) -> iq_line_3_6/1
  d_iq_load_5_block/1(Blockout_d_iq_load_5_f01ab) -> iq_load_5/1
  d_id_line_5_6_block/1(Blockout_d_id_line_5_6_b7e3f) -> id_line_5_6/1
  d_id_line_8_9_block/1(Blockout_d_id_line_8_9_12877) -> id_line_8_9/1
  d_id_load_5_block/1(Blockout_d_id_load_5_3ae5a) -> id_load_5/1
  d_id_load_9_block/1(Blockout_d_id_load_9_04629) -> id_load_9/1
  d_iq_line_1_4_block/1(Blockout_d_iq_line_1_4_15027) -> iq_line_1_4/1
  d_iq_line_4_5_block/1(Blockout_d_iq_line_4_5_800d2) -> iq_line_4_5/1
  d_vd_bus_2_block/1(Blockout_d_vd_bus_2_d1493) -> vd_bus_2/1
  d_iq_line_6_7_block/1(Blockout_d_iq_line_6_7_229ae) -> iq_line_6_7/1
  d_vq_bus_8_block/1(Blockout_d_vq_bus_8_3ee0b) -> vq_bus_8/1
  d_iq_line_8_9_block/1(Blockout_d_iq_line_8_9_05116) -> iq_line_8_9/1
  d_vq_bus_2_block/1(Blockout_d_vq_bus_2_cf3a3) -> vq_bus_2/1
  d_vd_bus_1_block/1(Blockout_d_vd_bus_1_5653c) -> vd_bus_1/1
  d_vq_bus_6_block/1(Blockout_d_vq_bus_6_3e8a8) -> vq_bus_6/1
  d_vd_bus_6_block/1(Blockout_d_vd_bus_6_439ef) -> vd_bus_6/1
  d_vd_bus_7_block/1(Blockout_d_vd_bus_7_1b5ff) -> vd_bus_7/1
  d_vd_bus_8_block/1(Blockout_d_vd_bus_8_dd61b) -> vd_bus_8/1
  d_vq_bus_5_block/1(Blockout_d_vq_bus_5_1eae7) -> vq_bus_5/1

== system case4/SG_D_1 ==
  v_d_SG_D_1 : Inport
  v_q_SG_D_1 : Inport  Port=2
  E_fd_SG_D_1 : Integrator  InitialCondition=2.036900823207848
  Px_1_SG_D_1 : Integrator  InitialCondition=0.0
  Px_2_SG_D_1 : Integrator  InitialCondition=0.0
  Px_3_SG_D_1 : Integrator  InitialCondition=-1.103223322171585e-24
  R_f_SG_D_1 : Integrator  InitialCondition=13.751990414971843
  T_e_SG_D_1_block : Subsystem
  T_m_SG_D_1 : Integrator  InitialCondition=0.7293159586498017
  V_f_SG_D_1 : Integrator  InitialCondition=20.36900823207848
  d_E_fd_SG_D_1_block : Subsystem
  d_Px_1_SG_D_1_block : Subsystem
  d_Px_2_SG_D_1_block : Subsystem
  d_Px_3_SG_D_1_block : Subsystem
  d_R_f_SG_D_1_block : Subsystem
  d_T_m_SG_D_1_block : Subsystem
  d_V_f_SG_D_1_block : Subsystem
  d_psi_1d_SG_D_1_block : Subsystem
  d_psi_d_SG_D_1_block : Subsystem
  d_psi_fd_SG_D_1_block : Subsystem
  d_psi_gq_SG_D_1_block : Subsystem
  d_psi_kq_SG_D_1_block : Subsystem
  d_psi_q_SG_D_1_block : Subsystem
  d_theta_SG_D_1_block : Subsystem
  d_w_SG_D_1_block : Subsystem
  i_d_SG_D_1_block : Subsystem
  i_q_SG_D_1_block : Subsystem
  psi_1d_SG_D_1 : Integrator  InitialCondition=0.8520566868605334
  psi_d_SG_D_1 : Integrator  InitialCondition=0.82003387236466
  psi_fd_SG_D_1 : Integrator  InitialCondition=1.013451671919735
  psi_gq_SG_D_1 : Integrator  InitialCondition=0.3530456355421974
  psi_kq_SG_D_1 : Integrator  InitialCondition=-0.5516338055346834
  psi_q_SG_D_1 : Integrator  InitialCondition=-0.5736991577560708
  theta_SG_D_1 : Integrator  InitialCondition=0.6101645693854417
  theta_SG_D_1_out_block : Subsystem
  w_SG_D_1 : Integrator  InitialCondition=376.99111843077515
  w_SG_D_1_out_block : Subsystem
  i_d_SG_D_1 : Outport
  i_q_SG_D_1 : Outport  Port=2
  T_e_SG_D_1 : Outport  Port=3
  w_SG_D_1_out : Outport  Port=4
  theta_SG_D_1_out : Outport  Port=5
  wires:
  V_f_SG_D_1/1 -> d_V_f_SG_D_1_block/14(State_V_f_SG_D_1_13f84), d_E_fd_SG_D_1_block/2(State_V_f_SG_D_1_5ae7d)
  psi_kq_SG_D_1/1 -> d_psi_q_SG_D_1_block/2(State_psi_kq_SG_D_1_6d221), d_psi_gq_SG_D_1_block/5(State_psi_kq_SG_D_1_ff60b), d_psi_gq_SG_D_1_block/8(State_psi_kq_SG_D_1_fd373), d_psi_kq_SG_D_1_block/2(State_psi_kq_SG_D_1_bc099), d_w_SG_D_1_block/5(State_psi_kq_SG_D_1_e3d67), d_psi_kq_SG_D_1_block/4(State_psi_kq_SG_D_1_a459f), i_d_SG_D_1_block/2(State_psi_kq_SG_D_1_27fd3), d_psi_gq_SG_D_1_block/3(State_psi_kq_SG_D_1_0b9ec), i_q_SG_D_1_block/2(State_psi_kq_SG_D_1_bf4f0), d_V_f_SG_D_1_block/10(State_psi_kq_SG_D_1_122aa), T_e_SG_D_1_block/3(State_psi_kq_SG_D_1_0d52f)
  w_SG_D_1_out_block/1(Blockout_w_SG_D_1_out_8a23b) -> w_SG_D_1_out/1
  d_theta_SG_D_1_block/1(Blockout_d_theta_SG_D_1_0ea3b) -> theta_SG_D_1/1
  d_Px_1_SG_D_1_block/1(Blockout_d_Px_1_SG_D_1_c0100) -> Px_1_SG_D_1/1
  w_SG_D_1/1 -> d_psi_q_SG_D_1_block/9(State_w_SG_D_1_ddf4d), d_w_SG_D_1_block/1(State_w_SG_D_1_a13c5), d_V_f_SG_D_1_block/8(State_w_SG_D_1_6da71), d_V_f_SG_D_1_block/13(State_w_SG_D_1_21a88), d_psi_d_SG_D_1_block/9(State_w_SG_D_1_d3493), d_Px_1_SG_D_1_block/2(State_w_SG_D_1_192b2), d_Px_2_SG_D_1_block/4(State_w_SG_D_1_8e384), d_theta_SG_D_1_block/1(State_w_SG_D_1_f434c), d_Px_3_SG_D_1_block/6(State_w_SG_D_1_924cf), w_SG_D_1_out_block/1(State_w_SG_D_1_a0747), d_T_m_SG_D_1_block/1(State_w_SG_D_1_428b2)
  d_T_m_SG_D_1_block/1(Blockout_d_T_m_SG_D_1_af57e) -> T_m_SG_D_1/1
  d_Px_2_SG_D_1_block/1(Blockout_d_Px_2_SG_D_1_bfa82) -> Px_2_SG_D_1/1
  d_Px_3_SG_D_1_block/1(Blockout_d_Px_3_SG_D_1_80a90) -> Px_3_SG_D_1/1
  d_E_fd_SG_D_1_block/1(Blockout_d_E_fd_SG_D_1_51614) -> E_fd_SG_D_1/1
  psi_1d_SG_D_1/1 -> d_psi_fd_SG_D_1_block/5(State_psi_1d_SG_D_1_4f731), d_psi_d_SG_D_1_block/1(State_psi_1d_SG_D_1_2ee34), d_w_SG_D_1_block/8(State_psi_1d_SG_D_1_a0c2c), d_V_f_SG_D_1_block/4(State_psi_1d_SG_D_1_11cfb), i_d_SG_D_1_block/5(State_psi_1d_SG_D_1_c944b), i_q_SG_D_1_block/5(State_psi_1d_SG_D_1_d0628), d_psi_1d_SG_D_1_block/3(State_psi_1d_SG_D_1_92ecb), d_psi_fd_SG_D_1_block/3(State_psi_1d_SG_D_1_08c92), d_psi_1d_SG_D_1_block/1(State_psi_1d_SG_D_1_22eb8), T_e_SG_D_1_block/6(State_psi_1d_SG_D_1_7d472), d_psi_fd_SG_D_1_block/8(State_psi_1d_SG_D_1_7ebda)
  Px_1_SG_D_1/1 -> d_Px_3_SG_D_1_block/5(State_Px_1_SG_D_1_97917), d_Px_2_SG_D_1_block/3(State_Px_1_SG_D_1_52394), d_Px_3_SG_D_1_block/4(State_Px_1_SG_D_1_408f6), d_Px_1_SG_D_1_block/1(State_Px_1_SG_D_1_9d70a), d_Px_2_SG_D_1_block/2(State_Px_1_SG_D_1_e74a6)
  T_m_SG_D_1/1 -> d_w_SG_D_1_block/2(State_T_m_SG_D_1_f43d2), d_T_m_SG_D_1_block/2(State_T_m_SG_D_1_d0a69)
  psi_q_SG_D_1/1 -> d_psi_d_SG_D_1_block/8(State_psi_q_SG_D_1_1479a), d_psi_q_SG_D_1_block/3(State_psi_q_SG_D_1_4ef79), d_psi_gq_SG_D_1_block/6(State_psi_q_SG_D_1_60255), d_psi_gq_SG_D_1_block/9(State_psi_q_SG_D_1_10770), d_psi_kq_SG_D_1_block/5(State_psi_q_SG_D_1_3b733), d_V_f_SG_D_1_block/7(State_psi_q_SG_D_1_c14d1), d_V_f_SG_D_1_block/11(State_psi_q_SG_D_1_9a2ac), d_w_SG_D_1_block/7(State_psi_q_SG_D_1_b5875), i_d_SG_D_1_block/3(State_psi_q_SG_D_1_7ff6d), i_q_SG_D_1_block/3(State_psi_q_SG_D_1_74a75), d_w_SG_D_1_block/6(State_psi_q_SG_D_1_2966f), T_e_SG_D_1_block/4(State_psi_q_SG_D_1_3dc92), T_e_SG_D_1_block/5(State_psi_q_SG_D_1_946b5)
  v_d_SG_D_1/1 -> d_psi_d_SG_D_1_block/4(Input_v_d_SG_D_1_2ca50), d_psi_q_SG_D_1_block/4(Input_v_d_SG_D_1_90d90)
  v_q_SG_D_1/1 -> d_psi_d_SG_D_1_block/6(Input_v_q_SG_D_1_1e814), d_psi_q_SG_D_1_block/6(Input_v_q_SG_D_1_a80c5)
  Px_2_SG_D_1/1 -> d_Px_3_SG_D_1_block/3(State_Px_2_SG_D_1_28cf3), d_Px_2_SG_D_1_block/1(State_Px_2_SG_D_1_e9b00), d_Px_3_SG_D_1_block/2(State_Px_2_SG_D_1_89bd0)
  psi_d_SG_D_1/1 -> d_psi_fd_SG_D_1_block/6(State_psi_d_SG_D_1_cb963), d_psi_fd_SG_D_1_block/9(State_psi_d_SG_D_1_ec3d5), d_psi_d_SG_D_1_block/2(State_psi_d_SG_D_1_3993f), d_psi_q_SG_D_1_block/8(State_psi_d_SG_D_1_9f1e2), d_w_SG_D_1_block/3(State_psi_d_SG_D_1_7f4c4), d_w_SG_D_1_block/9(State_psi_d_SG_D_1_f8ba7), d_V_f_SG_D_1_block/5(State_psi_d_SG_D_1_bfb9a), i_q_SG_D_1_block/6(State_psi_d_SG_D_1_d0c9d), d_psi_1d_SG_D_1_block/4(State_psi_d_SG_D_1_6d1a3), d_V_f_SG_D_1_block/12(State_psi_d_SG_D_1_510d3), T_e_SG_D_1_block/1(State_psi_d_SG_D_1_cf38e), T_e_SG_D_1_block/7(State_psi_d_SG_D_1_9ff9b), i_d_SG_D_1_block/6(State_psi_d_SG_D_1_499ff)
  theta_SG_D_1/1 -> d_psi_d_SG_D_1_block/5(State_theta_SG_D_1_ccf09), d_psi_q_SG_D_1_block/5(State_theta_SG_D_1_b8399), i_d_SG_D_1_block/4(State_theta_SG_D_1_c0d2f), d_psi_d_SG_D_1_block/7(State_theta_SG_D_1_4ed89), d_psi_q_SG_D_1_block/7(State_theta_SG_D_1_5aa7f), i_q_SG_D_1_block/8(State_theta_SG_D_1_20748), i_q_SG_D_1_block/4(State_theta_SG_D_1_baa8c), theta_SG_D_1_out_block/1(State_theta_SG_D_1_0c8fe), i_d_SG_D_1_block/8(State_theta_SG_D_1_3521f)
  psi_gq_SG_D_1/1 -> d_psi_q_SG_D_1_block/1(State_psi_gq_SG_D_1_fb8d0), d_psi_gq_SG_D_1_block/1(State_psi_gq_SG_D_1_6ef97), d_psi_gq_SG_D_1_block/2(State_psi_gq_SG_D_1_c0a1d), d_psi_gq_SG_D_1_block/4(State_psi_gq_SG_D_1_7636a), d_psi_gq_SG_D_1_block/7(State_psi_gq_SG_D_1_ba15c), d_w_SG_D_1_block/4(State_psi_gq_SG_D_1_23204), d_V_f_SG_D_1_block/9(State_psi_gq_SG_D_1_5ffd2), d_psi_kq_SG_D_1_block/3(State_psi_gq_SG_D_1_826db), i_d_SG_D_1_block/1(State_psi_gq_SG_D_1_d0d2e), i_q_SG_D_1_block/1(State_psi_gq_SG_D_1_2717f), d_psi_kq_SG_D_1_block/1(State_psi_gq_SG_D_1_29a0d), T_e_SG_D_1_block/2(State_psi_gq_SG_D_1_e3dd4)
  psi_fd_SG_D_1/1 -> d_psi_fd_SG_D_1_block/4(State_psi_fd_SG_D_1_d8d8e), d_psi_fd_SG_D_1_block/7(State_psi_fd_SG_D_1_e1815), d_psi_fd_SG_D_1_block/10(State_psi_fd_SG_D_1_d3425), d_psi_fd_SG_D_1_block/2(State_psi_fd_SG_D_1_0848f), d_psi_d_SG_D_1_block/3(State_psi_fd_SG_D_1_8a26a), d_psi_1d_SG_D_1_block/2(State_psi_fd_SG_D_1_06852), d_psi_1d_SG_D_1_block/5(State_psi_fd_SG_D_1_52850), d_V_f_SG_D_1_block/6(State_psi_fd_SG_D_1_57814), d_w_SG_D_1_block/10(State_psi_fd_SG_D_1_2ed74), i_q_SG_D_1_block/7(State_psi_fd_SG_D_1_58d0e), i_d_SG_D_1_block/7(State_psi_fd_SG_D_1_cd963), T_e_SG_D_1_block/8(State_psi_fd_SG_D_1_4d15b)
  d_V_f_SG_D_1_block/1(Blockout_d_V_f_SG_D_1_b8d13) -> V_f_SG_D_1/1
  d_R_f_SG_D_1_block/1(Blockout_d_R_f_SG_D_1_b6ceb) -> R_f_SG_D_1/1
  d_w_SG_D_1_block/1(Blockout_d_w_SG_D_1_60c3a) -> w_SG_D_1/1
  T_e_SG_D_1_block/1(Blockout_T_e_SG_D_1_a77ad) -> T_e_SG_D_1/1
  d_psi_q_SG_D_1_block/1(Blockout_d_psi_q_SG_D_1_390c6) -> psi_q_SG_D_1/1
  d_psi_d_SG_D_1_block/1(Blockout_d_psi_d_SG_D_1_83a0e) -> psi_d_SG_D_1/1
  i_q_SG_D_1_block/1(Blockout_i_q_SG_D_1_7a201) -> i_q_SG_D_1/1
  theta_SG_D_1_out_block/1(Blockout_theta_SG_D_1_out_ffb95) -> theta_SG_D_1_out/1
  d_psi_1d_SG_D_1_block/1(Blockout_d_psi_1d_SG_D_1_4f588) -> psi_1d_SG_D_1/1
  i_d_SG_D_1_block/1(Blockout_i_d_SG_D_1_645b0) -> i_d_SG_D_1/1
  d_psi_gq_SG_D_1_block/1(Blockout_d_psi_gq_SG_D_1_afee2) -> psi_gq_SG_D_1/1
  d_psi_kq_SG_D_1_block/1(Blockout_d_psi_kq_SG_D_1_c314f) -> psi_kq_SG_D_1/1
  R_f_SG_D_1/1 -> d_V_f_SG_D_1_block/2(State_R_f_SG_D_1_190e0), d_R_f_SG_D_1_block/2(State_R_f_SG_D_1_ef266)
  Px_3_SG_D_1/1 -> d_V_f_SG_D_1_block/3(State_Px_3_SG_D_1_49fda), d_Px_3_SG_D_1_block/1(State_Px_3_SG_D_1_45f45)
  E_fd_SG_D_1/1 -> d_V_f_SG_D_1_block/1(State_E_fd_SG_D_1_53fb1), d_R_f_SG_D_1_block/1(State_E_fd_SG_D_1_a2a74), d_E_fd_SG_D_1_block/1(State_E_fd_SG_D_1_c0e19), d_psi_fd_SG_D_1_block/1(State_E_fd_SG_D_1_29de2)
  d_psi_fd_SG_D_1_block/1(Blockout_d_psi_fd_SG_D_1_0294b) -> psi_fd_SG_D_1/1
